simulink library "Pressure_Drop_StorageHX"  (R2016b)
settings: Solver=ode45  StartTime=0.0  StopTime=10.0  RelTol=1e-3  EnableMultiTasking=on
libraries: carnot x3
settings Model: Creator=drhf  LastModifiedBy=drhf
settings DataIOCC: LimitDataPoints=on  SaveFormat=Array  SignalLoggingSaveFormat=ModelDataLogs
settings OptimizationCC: ExpressionDepthLimit=2147483647  LifeSpan=inf
settings DebuggingCC: UnderspecifiedInitializationDetection=Classic  MergeDetectMultiDrivingBlocksExec=none  SolverPrmCheckMsg=warning  FcnCallInpInsideContextMsg=warning  StateNameClashWarn=warning  SFUnexpectedBacktrackingDiag=warning  SFNoUnconditionalDefaultTransitionDiag=warning  SFExecutionAtInitializationDiag=none
settings HardwareCC: ProdBitPerPointer=32  ProdBitPerSizeT=32  ProdBitPerPtrDiffT=32  ProdLargestAtomicFloat=None  ProdIntDivRoundTo=Undefined  ProdEndianess=Unspecified  ProdWordSize=32  ProdHWDeviceType=32-bit Generic
settings ModelReferenceCC: PropagateSignalLabelsOutOfModel=off
settings GRTTargetCC: TargetLangStandard=C89/C90 (ANSI)  GeneratePreprocessorConditionals=Disable all  CombineOutputUpdateFcns=off  GRTInterface=on
settings ConfigComp: CovMetricSettings=dw  CovHtmlReporting=on  CovSaveCumulativeToWorkspaceVar=on  CovSaveSingleToWorkspaceVar=on  CovExternalEMLEnable=off

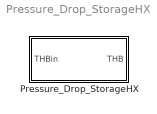
== system Pressure_Drop_StorageHX ==
  Pressure_Drop_StorageHX : Subsystem  mask(Pressure drop of tube heat exchanger in a storage){dia=1, hgt=1, dplin=10, dpqua=10}
      mask prompts: dia "Diameter of HX pipe [m]"; hgt "Height difference inlet-outlet [m]"; dplin "Pressure drop coefficient dplin [Pa/(kg/s)]"; dpqua "Pressure drop coefficient dpqua [Pa/(kg/s)²]"
      mask help:
      | Calculates the pressure drop in a tube heat exchanger according to:
      | dp = dpqua*mdot^2 + dplin*mdot + density*grav*height
      | with grav = 9.18 kg*m/s²
      mask Help: web(fullfile(path_carnot('help'),'Pressure_Drop_StorageHX.html'),'-helpbrowser')

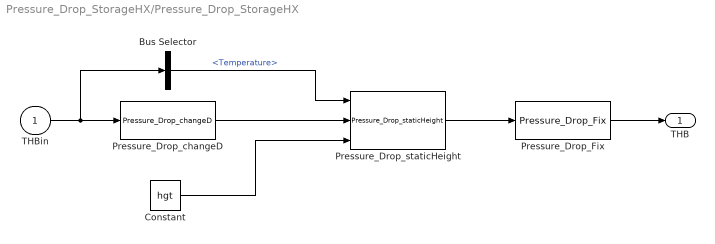
== system Pressure_Drop_StorageHX/Pressure_Drop_StorageHX ==
  THBin : Inport
  Bus Selector : BusSelector  OutputSignals=Temperature
  Constant : Constant  Value=hgt
  Pressure_Drop_Fix : carnot/Basic/Pressure_Drop/Pressure_Drop_Fix  con=0  lin=dplin  qua=dpqua
  Pressure_Drop_changeD : carnot/Basic/Pressure_Drop/Pressure_Drop_changeD  dia=dia
  Pressure_Drop_staticHeight : carnot/Basic/Pressure_Drop/Pressure_Drop_staticHeight
  THB : Outport
  wires:
  Pressure_Drop_Fix/1 -> THB/1
  Bus Selector/1 -> Pressure_Drop_staticHeight/1  "<Temperature>"
  THBin/1 -> Bus Selector/1, Pressure_Drop_changeD/1
  Constant/1 -> Pressure_Drop_staticHeight/3
  Pressure_Drop_changeD/1 -> Pressure_Drop_staticHeight/2
  Pressure_Drop_staticHeight/1 -> Pressure_Drop_Fix/1
